simulink model "multiportSwitch"  (R2022b)
settings: Solver=VariableStepAuto  StartTime=0.0  StopTime=10.0  MaxStep=1e-3  RelTol=1e-3
libraries: SignalEditorBlockLib x1
settings Model: Creator=bensweet  LastModifiedBy=bensweet
settings DebuggingCC: UnconnectedInputMsg=warning  UnconnectedOutputMsg=warning  UnconnectedLineMsg=warning
settings ModelReferenceCC: EnableRefExpFcnMdlSchedulingChecks=on
settings RTWCC: DLArmComputeVersion=19.05

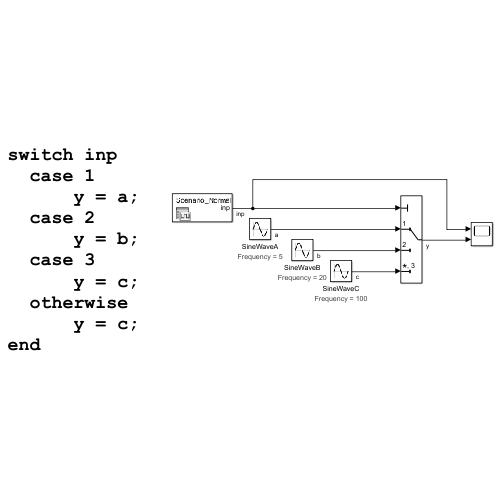
[thumbnail: Simulink's stored preview of the top-level diagram]
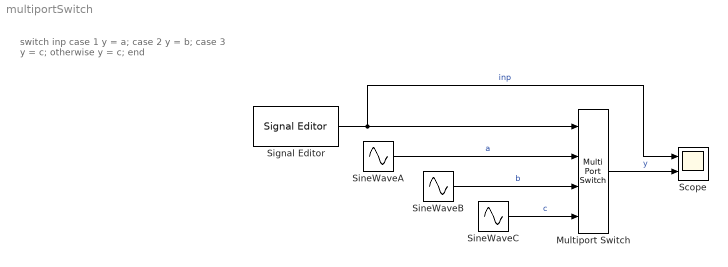
== system multiportSwitch ==
  note: switch inp
      | case 1
      | y = a;
      | case 2
      | y = b;
      | case 3
      | y = c;
      | otherwise
      | y = c;
      | end
  Multiport Switch : MultiPortSwitch  SaturateOnIntegerOverflow=off  InputSameDT=off
  Scope : Scope  NumInputPorts=2
  Signal Editor : SignalEditorBlockLib/Signal Editor  FileName=multiportSwitch_input.mat  ActiveScenario=Scenario_Normal  ActiveSignal=inp  IsBus=off  OutputBusObjectStr=Bus: BusObject  SampleTime=0  Interpolate=off  ZeroCross=off  OutputAfterFinalValue=Setting to zero  Unit=inherit  PreserveSignalName=on
  SineWaveA : Sin  Frequency=5  SampleTime=0
      settings: AttributesFormatString=Frequency = %<Frequency>
  SineWaveB : Sin  Frequency=20  SampleTime=0
      settings: AttributesFormatString=Frequency = %<Frequency>
  SineWaveC : Sin  Frequency=100  SampleTime=0
      settings: AttributesFormatString=Frequency = %<Frequency>
  wires:
  SineWaveA/1 -> Multiport Switch/2  "a"
  SineWaveB/1 -> Multiport Switch/3  "b"
  SineWaveC/1 -> Multiport Switch/4  "c"
  Signal Editor/1 -> Scope/1, Multiport Switch/1  "inp"
  Multiport Switch/1 -> Scope/2  "y"
